simulink model "lab1"  (R2017a)
settings: Solver=VariableStepAuto  StartTime=0.0  StopTime=10.0  RelTol=1e-3
settings Model: Creator=Mikle  LastModifiedBy=Mikle
settings DataIOCC: LimitDataPoints=on  SaveOutput=off  SaveTime=off
settings OptimizationCC: BlockReduction=off  BooleanDataType=off  LifeSpan=inf
settings DebuggingCC: SaveWithParameterizedLinksMsg=none  UnderspecifiedInitializationDetection=Classic  MergeDetectMultiDrivingBlocksExec=none  SignalResolutionControl=TryResolveAllWithWarning  AllowSymbolicDim=off  SFUnexpectedBacktrackingDiag=warning  SFNoUnconditionalDefaultTransitionDiag=warning  SFExecutionAtInitializationDiag=none
settings HardwareCC: TargetUnknown=on
settings GRTTargetCC: TargetLangStandard=C89/C90 (ANSI)  GeneratePreprocessorConditionals=Disable all

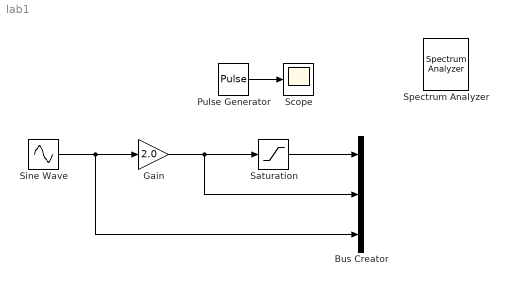
== system lab1 ==
  Bus Creator : BusCreator  Inputs=3
  Gain : Gain  Gain=2.0
  Pulse Generator : DiscretePulseGenerator  Period=10  PulseWidth=5
  Saturation : Saturate
  Scope : Scope
  Sine Wave : Sin  SineType=Sample based  SampleTime=0.1
  Spectrum Analyzer : SpectrumAnalyzer
  wires:
  Gain/1 -> Bus Creator/2, Saturation/1
  Sine Wave/1 -> Bus Creator/3, Gain/1
  Saturation/1 -> Bus Creator/1
  Pulse Generator/1 -> Scope/1
